simulink model "Longitudinal_fixed_slip"  (R2025b)
settings: Solver=VariableStepAuto  StartTime=0.0  StopTime=5  MaxStep=0.001  RelTol=1e-3
undefined symbols (not defined in the file): car, rad, s, Tau_1, Tau_2, Tau_3, Tau_4, Tau_EM, tyre
libraries: aerolibconvert2 x3, simulink x2
(part 1 of 2)
settings Model: Creator=mzacc  LastModifiedBy=loren

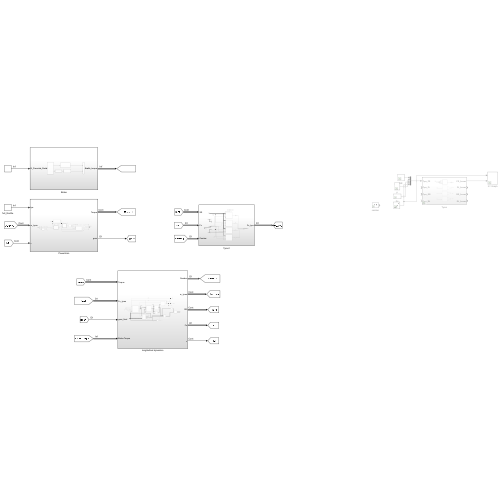
[thumbnail: Simulink's stored preview of the top-level diagram]
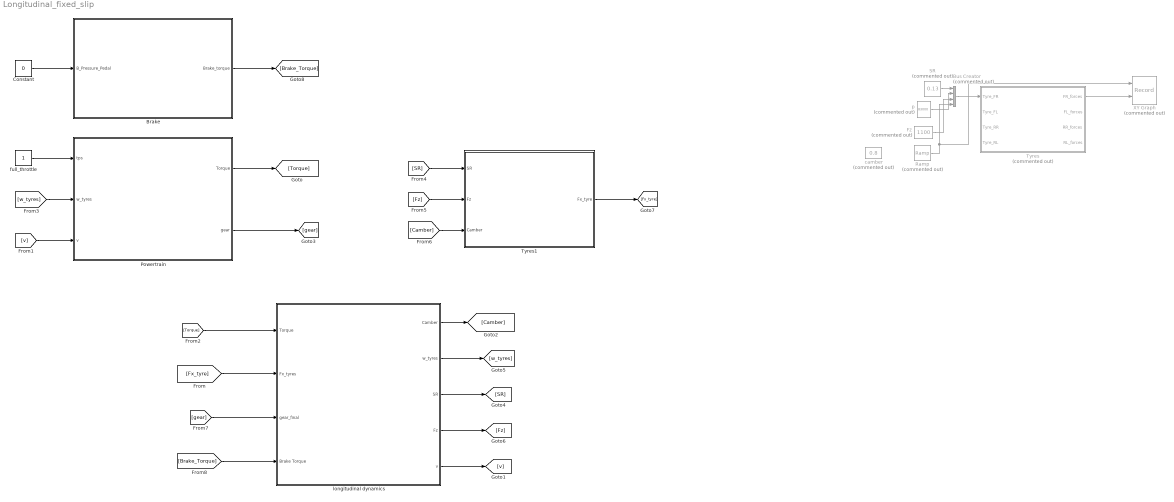
== system Longitudinal_fixed_slip ==
  Brake : Subsystem
  Bus Creator : BusCreator  Commented=on  Inputs=4
  Constant : Constant  Value=0
  Fz : Constant  Commented=on  Value=1100
  Powertrain : Subsystem
  Ramp : simulink/Sources/Ramp  Commented=on  slope=0.05  start=0  InitialOutput=-3
  SR : Constant  Commented=on  Value=0.13
  Tyres : Subsystem  Commented=on
  Tyres1 : Subsystem
  XY Graph : Record  Commented=on  NumPorts=2.0  FileSettingsInternal="{\"entries\":[{\"content\":{\"excelSettings\":{\"content\":{},\"type\":\"Streamout.ExcelSettings\"},\"parquetSettings\":{\"content\":{},\"type\":\"Streamout.ParquetSettings\"}},\"type\":\"Streamout.FileSettingStorage\",\"uuid\":\"\"}],\"packageUris\":[\"http:\\/\\/schema.mathworks.com\\/mf0\\/streamout_blocks\\/R2020a\"],\"version\":\"1.0\"}"  FrameSettings=[0, 0]  Layout=[1 1]  SignalsInternal="{\"entries\":[{\"content\":{},\"type\":\"RecordBlkView.InputSignals\",\"uuid\":\"\"}],\"packageUris\":[\"http:\\/\\/schema.mathworks.com\\/mf0\\/streamout_blocks\\/R2020a\"],\"version\":\"1.0\"}"  VisualizationBindings="{\"xyplotplugin\":{\"info\":[{\"series\":[],\"subplotID\":1}]}}"  CompatibilityTag=XY
  camber : Constant  Commented=on  Value=0.8
  full_throttle : Constant
  longitudinal dynamics : Subsystem
  p : Constant  Commented=on  Value=83000
  wires:
  [Fx_tyre] -> longitudinal dynamics/2(Fx_tyres)
  [Torque] -> longitudinal dynamics/1(Torque)
  Powertrain/1(Torque) -> [Torque]
  Fz/1 -> Bus Creator/3
  Tyres/1(FR_forces) -> XY Graph/2
  p/1 -> Bus Creator/2
  Bus Creator/1 -> Tyres/1(Tyre_FR)
  SR/1 -> Bus Creator/1
  Ramp/1 -> XY Graph/1, Bus Creator/4
  longitudinal dynamics/1(Camber) -> [Camber]
  [w_tyres] -> Powertrain/2(w_tyres)
  longitudinal dynamics/3(SR) -> [SR]
  longitudinal dynamics/2(w_tyres) -> [w_tyres]
  longitudinal dynamics/4(Fz) -> [Fz]
  longitudinal dynamics/5(v) -> [v]
  [v] -> Powertrain/3(v)
  [SR] -> Tyres1/1(SR)
  [Fz] -> Tyres1/2(Fz)
  [Camber] -> Tyres1/3(Camber)
  Tyres1/1(Fx_tyre) -> [Fx_tyre]
  full_throttle/1 -> Powertrain/1(tps)
  Powertrain/2(gear) -> [gear]
  [gear] -> longitudinal dynamics/3(gear_final)
  Constant/1 -> Brake/1(B_Pressure_Pedal)
  Brake/1(Brake_torque) -> [Brake_Torque]
  [Brake_Torque] -> longitudinal dynamics/4(Brake Torque)

== system Longitudinal_fixed_slip/Brake ==
  B_Pressure_Pedal : Inport
  Brake Balance : Subsystem
  Bus Creator : BusCreator  Inputs=2
  Front Caliper : Subsystem
  Proportioning Valve : Subsystem
  Rear Caliper : Subsystem
  Brake_torque : Outport
  wires:
  Brake Balance/1(P_Front) -> Front Caliper/1(P_Front)
  Proportioning Valve/1(p_rear_mod) -> Rear Caliper/1(P_rear)
  Brake Balance/2(P_rear) -> Proportioning Valve/1(P_rear)
  B_Pressure_Pedal/1 -> Brake Balance/1(Braking_Force)
  Bus Creator/1 -> Brake_torque/1
  Front Caliper/1(Brake_torque_front) -> Bus Creator/1  "Brake_torque_front"
  Rear Caliper/1(Brake_torque_rear) -> Bus Creator/2  "Brake_torque_rear"

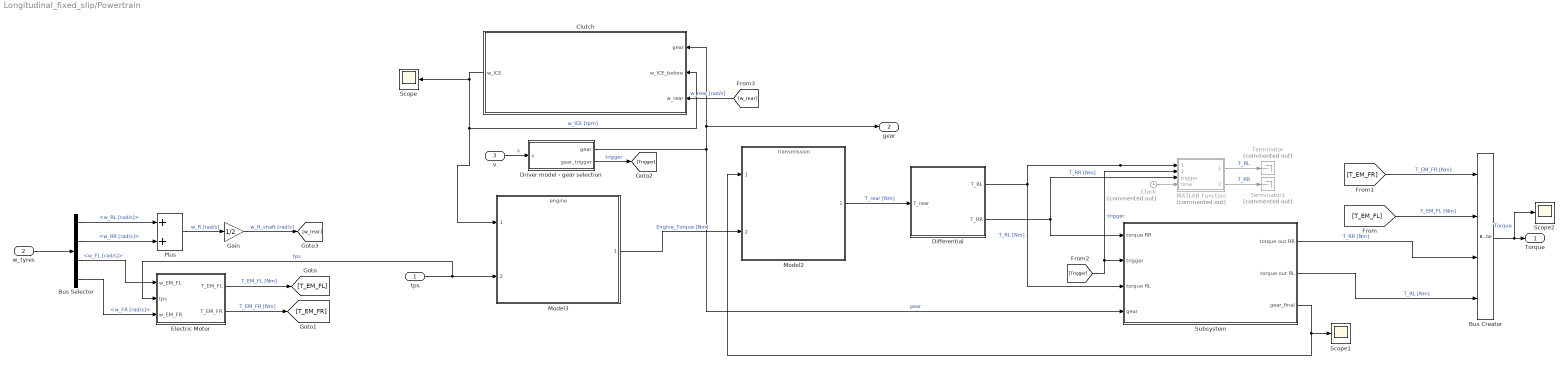
== system Longitudinal_fixed_slip/Powertrain ==
  tps : Inport
  w_tyres : Inport  Port=2
  v : Inport  Port=3
  Bus Creator : BusCreator  Inputs=4
  Bus Selector : BusSelector  OutputSignals=w_RL [rad/s],w_RR [rad/s],w_FL [rad/s],w_FR [rad/s]
  Clock : Clock  Commented=on
  Clutch : Subsystem
  Differential : Subsystem
  Driver model - gear selection : Subsystem
  Electric Motor : Subsystem
  Gain : Gain  Gain=1/2
  MATLAB Function : MATLAB Function  Commented=on  TreatAsAtomicUnit=on
  Model2 : ModelReference  ModelNameDialog=transmission.slx  SimulationMode=Normal  ModelReferenceVersion=3.11
  Model3 : ModelReference  ModelNameDialog=engine.slx  SimulationMode=Normal  ModelReferenceVersion=3.3
  Plus : Sum
  Scope : Scope
      settings: ActiveDisplayYMinimum=5410.5426113045514  ActiveDisplayYMaximum=8668.3318648594359  DataLoggingVariableName=ScopeData5
  Scope1 : Scope
      settings: ActiveDisplayYMinimum=-0.37499999999999989  ActiveDisplayYMaximum=3.375  DataLoggingVariableName=ScopeData4
  Scope2 : Scope
      settings: ActiveDisplayYMinimum=-45.581420561628825  ActiveDisplayYMaximum=410.23278505465947  DataLoggingVariableName=ScopeData19
  Subsystem : Subsystem
  Terminator : Terminator  Commented=on
  Terminator1 : Terminator  Commented=on
  Torque : Outport
  gear : Outport  Port=2
  wires:
  Model3/1 -> Model2/2  "Engine_Torque [Nm]"
  tps/1 -> Electric Motor/2(tps), Model3/2  "tps"
  Model2/1 -> Differential/1(T_rear)  "T_rear [Nm]"
  Bus Creator/1 -> Scope2/1, Torque/1  "Torque"
  Electric Motor/1(T_EM_FL) -> [T_EM_FL]  "T_EM_FL [Nm]"
  Electric Motor/2(T_EM_FR) -> [T_EM_FR]  "T_EM_FR [Nm]"
  [T_EM_FL] -> Bus Creator/2  "T_EM_FL [Nm]"
  [T_EM_FR] -> Bus Creator/1  "T_EM_FR [Nm]"
  Differential/2(T_RR) -> MATLAB Function/3(trigger), Subsystem/1(torque RR)  "T_RR [Nm]"
  Differential/1(T_RL) -> MATLAB Function/1(T_RL_in), Subsystem/3(torque RL)  "T_RL [Nm]"
  Driver model - gear selection/2(gear_trigger) -> [Trigger]  "trigger"
  [Trigger] -> MATLAB Function/2(T_RR_in), Subsystem/2(trigger)  "trigger"
  w_tyres/1 -> Bus Selector/1
  Bus Selector/1 -> Plus/1  "<w_RL [rad/s]>"
  Gain/1 -> [w_rear]  "w_R_shaft [rad/s]"
  Plus/1 -> Gain/1  "w_R [rad/s]"
  Driver model - gear selection/1(gear) -> gear/1, Clutch/1(gear), Subsystem/4(gear)  "gear"
  Clutch/1(w_ICE) -> Model3/1, Clutch/2(w_ICE_before), Scope/1  "w_ICE [rpm]"
  Bus Selector/2 -> Plus/2  "<w_RR [rad/s]>"
  Bus Selector/3 -> Electric Motor/1(w_EM_FL)  "<w_FL [rad/s]>"
  Bus Selector/4 -> Electric Motor/3(w_EM_FR)  "<w_FR [rad/s]>"
  [w_rear] -> Clutch/3(w_rear)  "w_rear [rad/s]"
  v/1 -> Driver model - gear selection/1(v)  "v"
  MATLAB Function/1(T_RL_out) -> Terminator/1  "T_RL"
  MATLAB Function/2(T_RR_out) -> Terminator1/1  "T_RR"
  Clock/1 -> MATLAB Function/4(time)
  Subsystem/1(torque out RR) -> Bus Creator/3  "T_RR [Nm]"
  Subsystem/2(torque out RL) -> Bus Creator/4  "T_RL [Nm]"
  Subsystem/3(gear_final) -> Scope1/1, Model2/1

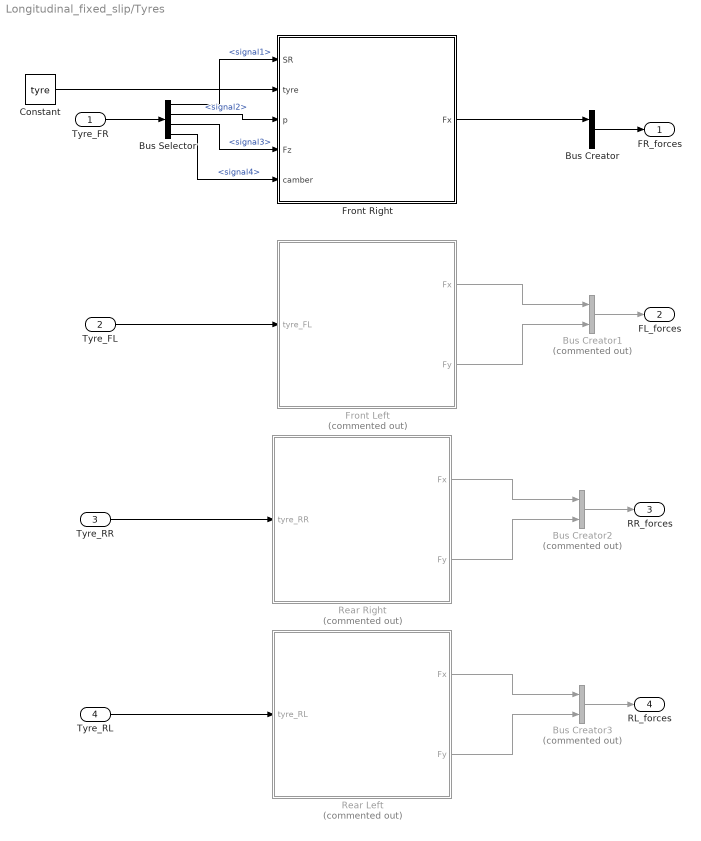
== system Longitudinal_fixed_slip/Tyres ==
  Tyre_FR : Inport
  Tyre_FL : Inport  Port=2
  Tyre_RR : Inport  Port=3
  Tyre_RL : Inport  Port=4
  Bus Creator : BusCreator  Inputs=2
  Bus Creator1 : BusCreator  Commented=on  Inputs=2
  Bus Creator2 : BusCreator  Commented=on  Inputs=2
  Bus Creator3 : BusCreator  Commented=on  Inputs=2
  Bus Selector : BusSelector  OutputSignals=signal1,signal2,signal3,signal4
  Constant : Constant  Value=tyre  OutDataTypeStr=Bus: slBus1
  Front Left : MATLAB Function  Commented=on  TreatAsAtomicUnit=on
  Front Right : MATLAB Function  TreatAsAtomicUnit=on
  Rear Left : MATLAB Function  Commented=on  TreatAsAtomicUnit=on
  Rear Right : MATLAB Function  Commented=on  TreatAsAtomicUnit=on
  FR_forces : Outport
  FL_forces : Outport  Port=2
  RR_forces : Outport  Port=3
  RL_forces : Outport  Port=4
  wires:
  Front Right/1(Fx) -> Bus Creator/1
  Tyre_FL/1 -> Front Left/1(tyre_FL)
  Tyre_RR/1 -> Rear Right/1(tyre_RR)
  Tyre_RL/1 -> Rear Left/1(tyre_RL)
  Bus Creator/1 -> FR_forces/1
  Front Left/1(Fx) -> Bus Creator1/1
  Front Left/2(Fy) -> Bus Creator1/2
  Bus Creator1/1 -> FL_forces/1
  Rear Right/1(Fx) -> Bus Creator2/1
  Rear Right/2(Fy) -> Bus Creator2/2
  Bus Creator2/1 -> RR_forces/1
  Rear Left/1(Fx) -> Bus Creator3/1
  Rear Left/2(Fy) -> Bus Creator3/2
  Bus Creator3/1 -> RL_forces/1
  Tyre_FR/1 -> Bus Selector/1
  Bus Selector/1 -> Front Right/1(SR)  "<signal1>"
  Bus Selector/2 -> Front Right/3(p)  "<signal2>"
  Bus Selector/3 -> Front Right/4(Fz)  "<signal3>"
  Bus Selector/4 -> Front Right/5(camber)  "<signal4>"
  Constant/1 -> Front Right/2(tyre)

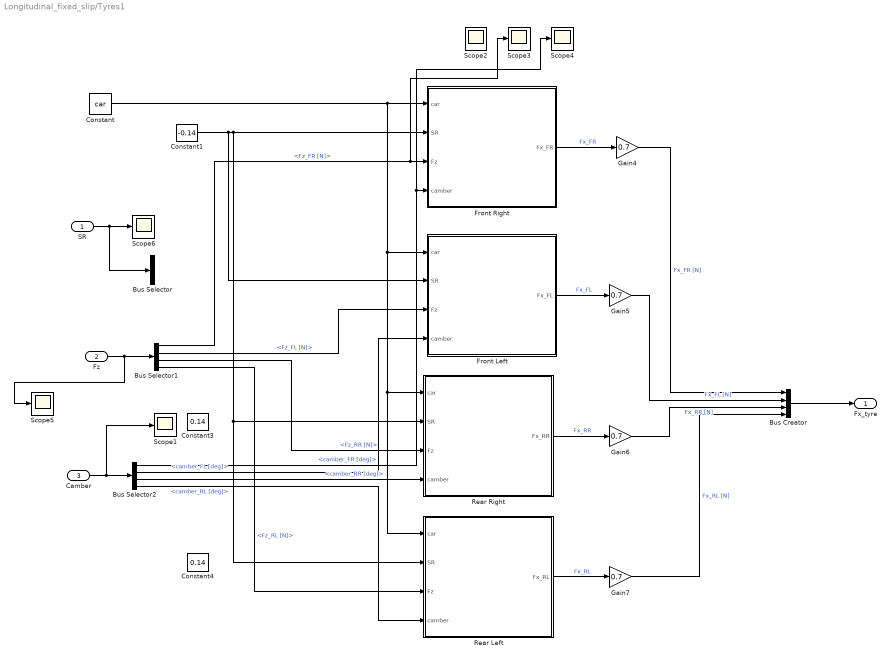
== system Longitudinal_fixed_slip/Tyres1 ==
  SR : Inport
  Fz : Inport  Port=2
  Camber : Inport  Port=3
  Bus Creator : BusCreator  Inputs=4
  Bus Selector : BusSelector  OutputSignals=SR_FL,SR_RL,SR_RR,SR_FR
  Bus Selector1 : BusSelector  OutputSignals=Fz_FR [N],Fz_FL [N],Fz_RR [N],Fz_RL [N]
  Bus Selector2 : BusSelector  OutputSignals=camber_FR [deg],camber_FL [deg],camber_RR [deg],camber_RL [deg]
  Constant : Constant  Value=car  OutDataTypeStr=Bus: slBus1
  Constant1 : Constant  Value=-0.14
  Constant3 : Constant  Value=0.14
  Constant4 : Constant  Value=0.14
  Front Left : MATLAB Function  TreatAsAtomicUnit=on
  Front Right : MATLAB Function  TreatAsAtomicUnit=on
  Gain{4..7} (4 alike) : Gain  Gain=0.7
  Rear Left : MATLAB Function  TreatAsAtomicUnit=on
  Rear Right : MATLAB Function  TreatAsAtomicUnit=on
  Scope{1..6} (6 alike) : Scope
      Scope1 settings: ActiveDisplayYMinimum=-1  ActiveDisplayYMaximum=1  DataLoggingVariableName=ScopeData27
      Scope2 settings: ActiveDisplayYMinimum=-1.2903982949278723  ActiveDisplayYMaximum=0.18800882212526682  DataLoggingVariableName=ScopeData6
      Scope3 settings: ActiveDisplayYMinimum=246.86785737661717  ActiveDisplayYMaximum=1297.36957232489  DataLoggingVariableName=ScopeData7
      Scope4 settings: ActiveDisplayYMinimum=-7.8867077725150958  ActiveDisplayYMaximum=2.0712522631883972  DataLoggingVariableName=ScopeData8
      Scope5 settings: ActiveDisplayYMinimum=-1  ActiveDisplayYMaximum=1  DataLoggingVariableName=ScopeData28
      Scope6 settings: ActiveDisplayYMinimum=-13.029799483705139  ActiveDisplayYMaximum=1.675400103949096  DataLoggingVariableName=ScopeData20
  Fx_tyre : Outport
  wires:
  Constant/1 -> Rear Left/1(car), Rear Right/1(car), Front Left/1(car), Front Right/1(car)
  Bus Creator/1 -> Fx_tyre/1
  Fz/1 -> Scope5/1, Bus Selector1/1
  Camber/1 -> Scope1/1, Bus Selector2/1
  Bus Selector1/1 -> Scope3/1, Front Right/3(Fz)  "<Fz_FR [N]>"
  Bus Selector2/1 -> Scope4/1, Front Right/4(camber)  "<camber_FR [deg]>"
  Bus Selector1/2 -> Front Left/3(Fz)  "<Fz_FL [N]>"
  Bus Selector1/3 -> Rear Right/3(Fz)  "<Fz_RR [N]>"
  Bus Selector1/4 -> Rear Left/3(Fz)  "<Fz_RL [N]>"
  Bus Selector2/2 -> Front Left/4(camber)  "<camber_FL [deg]>"
  Bus Selector2/3 -> Rear Right/4(camber)  "<camber_RR [deg]>"
  Bus Selector2/4 -> Rear Left/4(camber)  "<camber_RL [deg]>"
  SR/1 -> Bus Selector/1, Scope6/1
  Front Right/1(Fx_FR) -> Gain4/1  "Fx_FR"
  Front Left/1(Fx_FL) -> Gain5/1  "Fx_FL"
  Rear Right/1(Fx_RR) -> Gain6/1  "Fx_RR"
  Rear Left/1(Fx_RL) -> Gain7/1  "Fx_RL"
  Gain4/1 -> Bus Creator/1  "Fx_FR [N]"
  Gain5/1 -> Bus Creator/2  "Fx_FL [N]"
  Gain6/1 -> Bus Creator/3  "Fx_RR [N]"
  Gain7/1 -> Bus Creator/4  "Fx_RL [N]"
  Constant1/1 -> Rear Left/2(SR), Rear Right/2(SR), Front Right/2(SR), Front Left/2(SR)

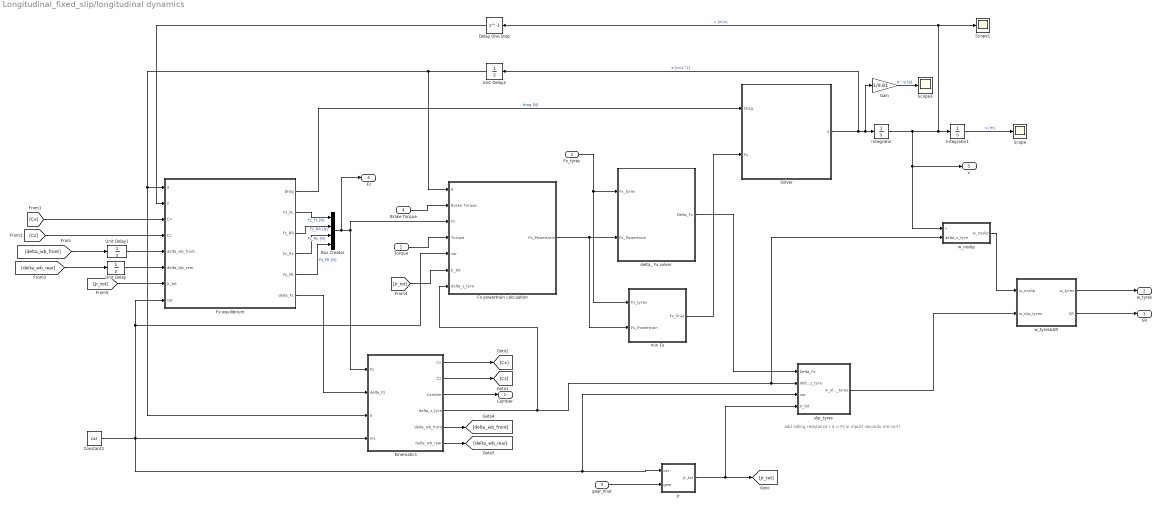
== system Longitudinal_fixed_slip/longitudinal dynamics ==
  note: add rolling resistance ( 4 = Fz in input) secondo me no!!!
  Torque : Inport
  Fx_tyres : Inport  Port=2
  gear_final : Inport  Port=3
  Brake Torque : Inport  Port=4
  Bus Creator : BusCreator  Inputs=4
  Constant1 : Constant  Value=car  OutDataTypeStr=Bus: slBus1
  Delay One Step : Delay  DelayLength=1
  Fx equilibrium : MATLAB Function  TreatAsAtomicUnit=on
  Fx powertrain calculation : Subsystem
  Gain : Gain  Gain=1/9.81
  Integrator : Integrator
  Integrator1 : Integrator
  Jr : Subsystem
  Kinematics : Subsystem
  Scope : Scope
      settings: ActiveDisplayYMinimum=2.4946310045593236  ActiveDisplayYMaximum=116.12903261010605
  Scope1 : Scope
      settings: ActiveDisplayYMinimum=-1  ActiveDisplayYMaximum=1
  Scope3 : Scope
      settings: ActiveDisplayYMinimum=-1.4648722058071688  ActiveDisplayYMaximum=0.89428927320913831  DataLoggingVariableName=ScopeData3
  Solver : Subsystem
  Unit Delay : UnitDelay  SampleTime=-1  HasFrameUpgradeWarning=on
  Unit Delay1 : UnitDelay  SampleTime=-1  HasFrameUpgradeWarning=on
  Unit Delay2 : UnitDelay  SampleTime=-1  HasFrameUpgradeWarning=on
  delta_ Fx solver : Subsystem
  min Fx : Subsystem
  slip_tyres : Subsystem
  w_noslip : Subsystem
  w_tyres&SR : Subsystem
  Camber : Outport
  w_tyres : Outport  Port=2
  SR : Outport  Port=3
  Fz : Outport  Port=4
  v : Outport  Port=5
  wires:
  Torque/1 -> Fx powertrain calculation/4(Torque)
  Integrator1/1 -> Scope/1  "s [m]"
  Integrator/1 -> Delay One Step/1, Scope1/1, Integrator1/1, w_noslip/1(v), v/1  "v [m/s]"
  Fx equilibrium/2(Fz_FL) -> Bus Creator/1  "Fz_FL [N]"
  Fx equilibrium/3(Fz_RR) -> Bus Creator/2  "Fz_RR [N]"
  Fx equilibrium/4(Fz_RL) -> Bus Creator/3  "Fz_RL [N]"
  Fx equilibrium/5(Fz_FR) -> Bus Creator/4  "Fz_FR [N]"
  Bus Creator/1 -> Fz/1, Kinematics/1(Fz), Fx powertrain calculation/3(Fz)
  Fx powertrain calculation/1(Fx_Powertrain) -> min Fx/2(Fx_Powertrain), delta_ Fx solver/2(Fx_Powertrain)
  Fx_tyres/1 -> min Fx/1(Fx_tyres), delta_ Fx solver/1(Fx_tyres)
  delta_ Fx solver/1(Delta_Fx) -> slip_tyres/1(Delta_Fx)
  Kinematics/4(delta_z_tyre) -> Fx powertrain calculation/7(delta_z_tyre), w_noslip/2(delta_z_tyre), slip_tyres/2(delta_z_tyre)
  Kinematics/3(Camber) -> Camber/1
  slip_tyres/1(w_slip_tyres) -> w_tyres&SR/2(w_slip_tyres)
  Fx equilibrium/6(delta_Fz) -> Kinematics/2(delta_Fz)
  Kinematics/2(Cz) -> [Cz]
  Kinematics/1(Cx) -> [Cx]
  [Cx] -> Fx equilibrium/3(Cx)
  [Cz] -> Fx equilibrium/4(Cz)
  Kinematics/5(delta_wb_front) -> [delta_wb_front]
  Kinematics/6(delta_wb_rear) -> [delta_wb_rear]
  [delta_wb_front] -> Unit Delay1/1
  [delta_wb_rear] -> Unit Delay/1
  w_tyres&SR/1(w_tyres) -> w_tyres/1
  w_tyres&SR/2(SR) -> SR/1
  Fx equilibrium/1(Drag) -> Solver/1(Drag)  "drag [N]"
  Delay One Step/1 -> Fx equilibrium/2(v)
  Unit Delay2/1 -> Fx powertrain calculation/1(a), Kinematics/3(a), Fx equilibrium/1(a)
  Constant1/1 -> Jr/1(car), slip_tyres/3(car), Kinematics/4(In1), Fx powertrain calculation/5(car), Fx equilibrium/8(car)
  Unit Delay1/1 -> Fx equilibrium/5(delta_wb_front)
  Solver/1(a) -> Unit Delay2/1, Gain/1, Integrator/1  "a [m/s^2]"
  Gain/1 -> Scope3/1  "a - g [g]"
  w_noslip/1(w_noslip) -> w_tyres&SR/1(w_noslip)
  Unit Delay/1 -> Fx equilibrium/6(delta_wb_rear)
  gear_final/1 -> Jr/2(gear)
  Jr/1(Jr_tot) -> [Jr_tot], slip_tyres/4(Jr_tot)
  [Jr_tot] -> Fx powertrain calculation/6(Jr_tot)
  [Jr_tot] -> Fx equilibrium/7(Jr_tot)
  Brake Torque/1 -> Fx powertrain calculation/2(Brake Torque)
  min Fx/1(Fx_final) -> Solver/2(Fx)

== system Longitudinal_fixed_slip/Brake/Brake Balance ==
  Braking_Force : Inport
  1- Brake_Balance : Gain  Gain=1-car.brakebalance
  Brake_Balance : Gain  Gain=car.brakebalance
  P_Front : Outport
  P_rear : Outport  Port=2
  wires:
  Braking_Force/1 -> Brake_Balance/1, 1- Brake_Balance/1
  1- Brake_Balance/1 -> P_rear/1  "P_rear"
  Brake_Balance/1 -> P_Front/1  "P_Front"

== system Longitudinal_fixed_slip/Brake/Front Caliper ==
  P_Front : Inport
  Gain : Gain  Gain=4
  Pad Friction : Gain  Gain=car.brakepad_friction_coeff
  Piston Area : Gain  Gain=pi*(car.brakepistondiameter)^2/4
  brake radius : Gain  Gain=car.brake_radius_front
  Brake_torque_front : Outport
  wires:
  P_Front/1 -> Gain/1
  Gain/1 -> Piston Area/1
  Piston Area/1 -> Pad Friction/1
  Pad Friction/1 -> brake radius/1
  brake radius/1 -> Brake_torque_front/1

== system Longitudinal_fixed_slip/Brake/Proportioning Valve ==
  P_rear : Inport
  Saturation : Saturate  UpperLimit=car.proportioning_valve_cutting_p  LowerLimit=0
  p_rear_mod : Outport
  wires:
  Saturation/1 -> p_rear_mod/1
  P_rear/1 -> Saturation/1

== system Longitudinal_fixed_slip/Brake/Rear Caliper ==
  P_rear : Inport
  Gain : Gain  Gain=2
  Pad Friction : Gain  Gain=car.brakepad_friction_coeff
  Piston Area : Gain  Gain=pi*(car.brakepistondiameter)^2/4
  brake radius_rear : Gain  Gain=car.brake_radius_rear
  Brake_torque_rear : Outport
  wires:
  Piston Area/1 -> Pad Friction/1
  Gain/1 -> Piston Area/1
  P_rear/1 -> Gain/1
  Pad Friction/1 -> brake radius_rear/1
  brake radius_rear/1 -> Brake_torque_rear/1

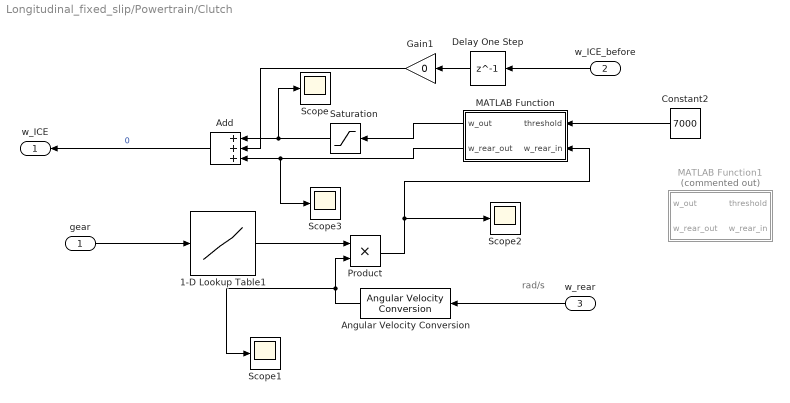
== system Longitudinal_fixed_slip/Powertrain/Clutch ==
  note: rad/s
  gear : Inport
  w_ICE_before : Inport  Port=2
  w_rear : Inport  Port=3
  1-D Lookup Table1 : Lookup_n-D  NumberOfTableDimensions=1  BreakpointsForDimension1=[1;2;3;4]  Table=[Tau_1; Tau_2; Tau_3; Tau_4]  InternalRulePriority=Speed  RndMeth=Simplest
  Add : Sum  Inputs=+++
  Angular Velocity Conversion : aerolibconvert2/Angular Velocity Conversion  IU=rad/s  OU=rpm
  Constant2 : Constant  Value=7000
  Delay One Step : Delay  DelayLength=1
  Gain1 : Gain  Gain=0
  MATLAB Function : MATLAB Function  TreatAsAtomicUnit=on  SystemSampleTime=0.001
  MATLAB Function1 : MATLAB Function  Commented=on  TreatAsAtomicUnit=on  SystemSampleTime=0.001
  Product : Product
  Saturation : Saturate  UpperLimit=10000  LowerLimit=0
  Scope{,1..3} (4 alike) : Scope
      Scope settings: ActiveDisplayYMinimum=-2311.872852964088  ActiveDisplayYMaximum=5444.7682269284924  DataLoggingVariableName=ScopeData9
      Scope1 settings: ActiveDisplayYMinimum=-1  ActiveDisplayYMaximum=1  DataLoggingVariableName=ScopeData16
      Scope2 settings: ActiveDisplayYMinimum=-1232.0255145373203  ActiveDisplayYMaximum=15203.537686190353  DataLoggingVariableName=ScopeData22
      Scope3 settings: ActiveDisplayYMinimum=-5859.3618694424358  ActiveDisplayYMaximum=14721.316107465498  DataLoggingVariableName=ScopeData23
  w_ICE : Outport
  wires:
  Saturation/1 -> Scope/1, Add/1
  MATLAB Function/1(w_out) -> Saturation/1
  w_rear/1 -> Angular Velocity Conversion/1
  1-D Lookup Table1/1 -> Product/1
  Product/1 -> Scope2/1, MATLAB Function/2(w_rear_in)
  Delay One Step/1 -> Gain1/1
  w_ICE_before/1 -> Delay One Step/1
  gear/1 -> 1-D Lookup Table1/1
  Gain1/1 -> Add/2
  Add/1 -> w_ICE/1  "0"
  Angular Velocity Conversion/1 -> Scope1/1, Product/2
  Constant2/1 -> MATLAB Function/1(threshold)
  MATLAB Function/2(w_rear_out) -> Scope3/1, Add/3

== system Longitudinal_fixed_slip/Powertrain/Differential ==
  T_rear : Inport
  Gain : Gain  Gain=0.5
  T_RL : Outport
  T_RR : Outport  Port=2
  wires:
  T_rear/1 -> Gain/1
  Gain/1 -> T_RR/1, T_RL/1

== system Longitudinal_fixed_slip/Powertrain/Driver model - gear selection ==
  v : Inport
  Constant : Constant  Value=car  OutDataTypeStr=Bus: slBus1
  MATLAB Function3 : MATLAB Function  TreatAsAtomicUnit=on
  gear : Outport
  gear_trigger : Outport  Port=2
  wires:
  MATLAB Function3/2(gear_out) -> gear/1
  MATLAB Function3/1(gear_trigger) -> gear_trigger/1  "trigger"
  v/1 -> MATLAB Function3/2(v)
  Constant/1 -> MATLAB Function3/1(car)

== system Longitudinal_fixed_slip/Powertrain/Electric Motor ==
  w_EM_FL : Inport
  tps : Inport  Port=2
  w_EM_FR : Inport  Port=3
  2-D Lookup Table : Lookup_n-D  BreakpointsForDimension1=[0;5415.9399999999996;5455.8699999999999;5494.6300000000001;5524.8000000000002;5801.2200000000003;6194.8599999999997;6620.2799999999997;6996.5;7478.6599999999999;8072.5500000000002;8891.9799999999996;8998.9200000000001;9966.8600000000006;10994.200000000001;11872.6;13016.16;13972.65;15994.85]  BreakpointsForDimension2=[0;0.25;0.29999999999999999;0.34999999999999998;0.40000000000000002;0.45000000000000001;0.5;0.59999999999999998;0.69999999999999996;0.80000000000000004;1]  Table=[0 1.72854705 2.07425646 2.41996587 2.7656752899999999 3.1113846999999999 3.4570941099999999 4.1485129299999999 4.8399317000000002 5.5313505699999999 6.9141880000000002;0 1.72755429 2.0730651500000001 2.4185760100000002 2.7640868599999999 3.10959772 3.4551085800000001 4.1461303000000003 4.8371519999999997 5.5281737299999998 6.9102170000000003;0 1.7172173399999999 2.0606608099999999 2.4041042799999999 2.7475477499999998 3.0909912099999999 3.4344346799999999 4.1213216199999998 4.8082086000000004 5.4950954899999997 6.8688690000000001;0 1.7114327 2.0537192399999999 2.3960057799999999 2.7382923199999998 3.0805788600000001 3.4228654000000001 4.1074384799999999 4.7920116000000004 5.4765846399999996 6.8457309999999998;0 1.7057860899999999 2.0469433100000001 2.3881005200000001 2.72925774 3.0704149599999999 3.4115721799999998 4.0938866100000002 4.7762010000000004 5.45851548 6.8231440000000001;0 1.65353861 1.9842463299999999 2.3149540499999999 2.6456617699999998 2.9763694900000002 3.3070772100000001 3.96849265 4.6299080999999997 5.2913235399999996 6.6141540000000001;0 1.57836584 1.89403901 2.2097121799999999 2.5253853500000001 2.8410585199999998 3.15673168 3.7880780199999999 4.4194243999999996 5.0507707000000002 6.3134629999999996;0 1.5001957400000001 1.80023489 2.10027404 2.4003131899999999 2.7003523399999998 3.0003914800000002 3.6004697800000001 4.2005480999999998 4.8006263699999998 6.0007830000000002;0 1.43080228 1.71696274 2.0031231900000002 2.2892836499999998 2.5754440999999999 2.86160456 3.4339254700000001 4.0062464000000002 4.5785672899999996 5.7232089999999998;0 1.34976662 1.6197199499999999 1.8896732700000001 2.1596266000000002 2.4295799200000001 2.69953325 3.2394398899999999 3.7793464999999999 4.3192531900000004 5.3990660000000004;0 1.24874098 1.49848917 1.74823737 1.99798556 2.24773376 2.4974819500000001 2.9969783400000001 3.4964746999999998 3.9959711200000001 4.9949640000000004;0 1.1245459799999999 1.3494551800000001 1.57436438 1.79927357 2.0241827699999999 2.2490919699999998 2.6989103600000002 3.1487288000000002 3.5985471499999999 4.4981840000000002;0 1.11256427 1.3350771299999999 1.5575899799999999 1.7801028299999999 2.0026156899999998 2.22512854 2.67015425 3.1151800000000001 3.5602056700000002 4.4502569999999997;0 0.98525799000000003 1.18230959 1.3793611800000001 1.5764127800000001 1.7734643800000001 1.9705159800000001 2.3646191700000001 2.7587223999999999 3.1528255600000001 3.9410319999999999;0 0.88127745999999996 1.0575329600000001 1.23378845 1.41004394 1.5862994399999999 1.7625549300000001 2.1150659100000002 2.4675769000000001 2.8200878899999999 3.5251100000000002;0 0.79965012999999996 0.95958014999999997 1.11951018 1.2794402 1.43937023 1.59930025 1.9191602999999999 2.2390203999999998 2.5588804000000001 3.198601;0 0.70417978000000003 0.84501572999999996 0.98585168999999995 1.1266876400000001 1.2675236000000001 1.4083595600000001 1.6900314700000001 1.9717034 2.2533752900000001 2.816719;0 0.63972525999999996 0.76767032000000002 0.89561537000000002 1.0235604199999999 1.15150547 1.2794505300000001 1.5353406300000001 1.7912307000000001 2.0471208399999998 2.5589010000000001;0 0.51010575999999996 0.61212690999999997 0.71414805999999997 0.81616922000000003 0.91819037000000003 1.0202115199999999 1.2242538199999999 1.4282961000000001 1.6323384299999999 2.0404230000000001]  InternalRulePriority=Speed  RndMeth=Simplest
      settings: InputPortMap=u0,u1
  2-D Lookup Table1 : Lookup_n-D  BreakpointsForDimension1=[0;5415.9399999999996;5455.8699999999999;5494.6300000000001;5524.8000000000002;5801.2200000000003;6194.8599999999997;6620.2799999999997;6996.5;7478.6599999999999;8072.5500000000002;8891.9799999999996;8998.9200000000001;9966.8600000000006;10994.200000000001;11872.6;13016.16;13972.65;15994.85]  BreakpointsForDimension2=[0;0.25;0.29999999999999999;0.34999999999999998;0.40000000000000002;0.45000000000000001;0.5;0.59999999999999998;0.69999999999999996;0.80000000000000004;1]  Table=[0 1.72854705 2.07425646 2.41996587 2.7656752899999999 3.1113846999999999 3.4570941099999999 4.1485129299999999 4.8399317000000002 5.5313505699999999 6.9141880000000002;0 1.72755429 2.0730651500000001 2.4185760100000002 2.7640868599999999 3.10959772 3.4551085800000001 4.1461303000000003 4.8371519999999997 5.5281737299999998 6.9102170000000003;0 1.7172173399999999 2.0606608099999999 2.4041042799999999 2.7475477499999998 3.0909912099999999 3.4344346799999999 4.1213216199999998 4.8082086000000004 5.4950954899999997 6.8688690000000001;0 1.7114327 2.0537192399999999 2.3960057799999999 2.7382923199999998 3.0805788600000001 3.4228654000000001 4.1074384799999999 4.7920116000000004 5.4765846399999996 6.8457309999999998;0 1.7057860899999999 2.0469433100000001 2.3881005200000001 2.72925774 3.0704149599999999 3.4115721799999998 4.0938866100000002 4.7762010000000004 5.45851548 6.8231440000000001;0 1.65353861 1.9842463299999999 2.3149540499999999 2.6456617699999998 2.9763694900000002 3.3070772100000001 3.96849265 4.6299080999999997 5.2913235399999996 6.6141540000000001;0 1.57836584 1.89403901 2.2097121799999999 2.5253853500000001 2.8410585199999998 3.15673168 3.7880780199999999 4.4194243999999996 5.0507707000000002 6.3134629999999996;0 1.5001957400000001 1.80023489 2.10027404 2.4003131899999999 2.7003523399999998 3.0003914800000002 3.6004697800000001 4.2005480999999998 4.8006263699999998 6.0007830000000002;0 1.43080228 1.71696274 2.0031231900000002 2.2892836499999998 2.5754440999999999 2.86160456 3.4339254700000001 4.0062464000000002 4.5785672899999996 5.7232089999999998;0 1.34976662 1.6197199499999999 1.8896732700000001 2.1596266000000002 2.4295799200000001 2.69953325 3.2394398899999999 3.7793464999999999 4.3192531900000004 5.3990660000000004;0 1.24874098 1.49848917 1.74823737 1.99798556 2.24773376 2.4974819500000001 2.9969783400000001 3.4964746999999998 3.9959711200000001 4.9949640000000004;0 1.1245459799999999 1.3494551800000001 1.57436438 1.79927357 2.0241827699999999 2.2490919699999998 2.6989103600000002 3.1487288000000002 3.5985471499999999 4.4981840000000002;0 1.11256427 1.3350771299999999 1.5575899799999999 1.7801028299999999 2.0026156899999998 2.22512854 2.67015425 3.1151800000000001 3.5602056700000002 4.4502569999999997;0 0.98525799000000003 1.18230959 1.3793611800000001 1.5764127800000001 1.7734643800000001 1.9705159800000001 2.3646191700000001 2.7587223999999999 3.1528255600000001 3.9410319999999999;0 0.88127745999999996 1.0575329600000001 1.23378845 1.41004394 1.5862994399999999 1.7625549300000001 2.1150659100000002 2.4675769000000001 2.8200878899999999 3.5251100000000002;0 0.79965012999999996 0.95958014999999997 1.11951018 1.2794402 1.43937023 1.59930025 1.9191602999999999 2.2390203999999998 2.5588804000000001 3.198601;0 0.70417978000000003 0.84501572999999996 0.98585168999999995 1.1266876400000001 1.2675236000000001 1.4083595600000001 1.6900314700000001 1.9717034 2.2533752900000001 2.816719;0 0.63972525999999996 0.76767032000000002 0.89561537000000002 1.0235604199999999 1.15150547 1.2794505300000001 1.5353406300000001 1.7912307000000001 2.0471208399999998 2.5589010000000001;0 0.51010575999999996 0.61212690999999997 0.71414805999999997 0.81616922000000003 0.91819037000000003 1.0202115199999999 1.2242538199999999 1.4282961000000001 1.6323384299999999 2.0404230000000001]  InternalRulePriority=Speed  RndMeth=Simplest
      settings: InputPortMap=u0,u1
  Angular Velocity Conversion : aerolibconvert2/Angular Velocity Conversion  IU=rad/s  OU=rpm
  Angular Velocity Conversion1 : aerolibconvert2/Angular Velocity Conversion  IU=rad/s  OU=rpm
  Gain{,1..3} (4 alike) : Gain  Gain=Tau_EM
  Limiter : Saturate  UpperLimit=16000  LowerLimit=0
  Limiter1 : Saturate  UpperLimit=16000  LowerLimit=0
  T_EM_FL : Outport
  T_EM_FR : Outport  Port=2
  wires:
  2-D Lookup Table/1 -> Gain/1
  Gain1/1 -> T_EM_FR/1
  2-D Lookup Table1/1 -> Gain1/1
  Gain/1 -> T_EM_FL/1
  Limiter/1 -> 2-D Lookup Table/1
  Limiter1/1 -> 2-D Lookup Table1/1
  tps/1 -> 2-D Lookup Table1/2, 2-D Lookup Table/2
  w_EM_FL/1 -> Angular Velocity Conversion/1
  w_EM_FR/1 -> Angular Velocity Conversion1/1
  Angular Velocity Conversion/1 -> Gain2/1
  Gain2/1 -> Limiter/1
  Angular Velocity Conversion1/1 -> Gain3/1
  Gain3/1 -> Limiter1/1

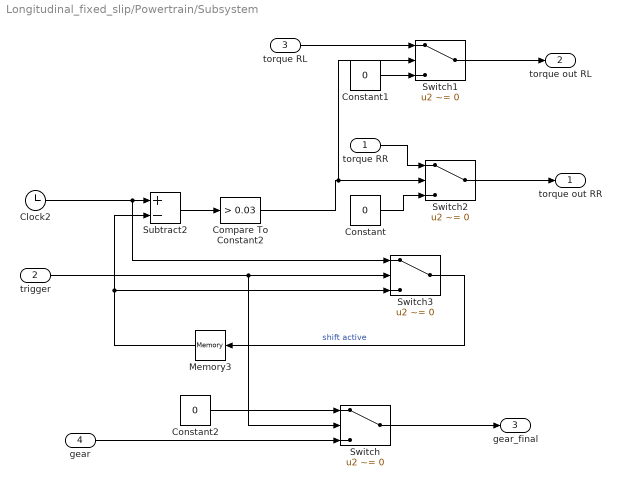
== system Longitudinal_fixed_slip/Powertrain/Subsystem ==
  torque RR : Inport
  trigger : Inport  Port=2
  torque RL : Inport  Port=3
  gear : Inport  Port=4
  Clock2 : Clock
  Compare To Constant2 : simulink/Logic and Bit Operations/Compare To Constant  relop=>  const=0.03  OutDataTypeStr=boolean
  Constant : Constant  Value=0
  Constant1 : Constant  Value=0
  Constant2 : Constant  Value=0
  Memory3 : Memory  InitialCondition=-0.1
  Subtract2 : Sum  Inputs=+-
  Switch{,1..3} (4 alike) : Switch  Criteria=u2 ~= 0  SaturateOnIntegerOverflow=off  InputSameDT=off
  torque out RR : Outport
  torque out RL : Outport  Port=2
  gear_final : Outport  Port=3
  wires:
  Memory3/1 -> Switch3/3, Subtract2/2
  trigger/1 -> Switch/2, Switch3/2
  Switch3/1 -> Memory3/1  "shift active"
  Subtract2/1 -> Compare To Constant2/1
  Switch2/1 -> torque out RR/1
  Switch1/1 -> torque out RL/1
  torque RR/1 -> Switch2/1
  Constant/1 -> Switch2/3
  Constant1/1 -> Switch1/3
  torque RL/1 -> Switch1/1
  Compare To Constant2/1 -> Switch1/2, Switch2/2
  Clock2/1 -> Switch3/1, Subtract2/1
  Constant2/1 -> Switch/1
  gear/1 -> Switch/3
  Switch/1 -> gear_final/1

== system Longitudinal_fixed_slip/longitudinal dynamics/Fx powertrain calculation ==
  a : Inport
  Brake Torque : Inport  Port=2
  Fz : Inport  Port=3
  Torque : Inport  Port=4
  car : Inport  Port=5
  Jr_tot : Inport  Port=6
  delta_z_tyre : Inport  Port=7
  Bus Creator : BusCreator  Inputs=4
  Bus Selector : BusSelector  OutputSignals=T_EM_FL [Nm],T_RR [Nm],T_EM_FR [Nm],T_RL [Nm]
  Bus Selector1 : BusSelector  OutputSignals=Fz_FL [N],Fz_RR [N],Fz_FR [N],Fz_RL [N]
  Bus Selector2 : BusSelector  OutputSignals=Brake_torque_front,Brake_torque_rear
  Bus Selector3 : BusSelector  OutputSignals=delta_z_tyre_FL,delta_z_tyre_RR,delta_z_tyre_FR,delta_z_tyre_RL
  FL : MATLAB Function  TreatAsAtomicUnit=on
  FR : MATLAB Function  TreatAsAtomicUnit=on
  RL : MATLAB Function  TreatAsAtomicUnit=on
  RR : MATLAB Function  TreatAsAtomicUnit=on
  Fx_Powertrain : Outport
  wires:
  FL/1(Fx_EM_FL) -> Bus Creator/1
  RR/1(Fx_ICE_RR) -> Bus Creator/2
  FR/1(Fx_EM_FR) -> Bus Creator/3
  Bus Creator/1 -> Fx_Powertrain/1
  RL/1(Fx_ICE_RL) -> Bus Creator/4
  Torque/1 -> Bus Selector/1
  Bus Selector/1 -> FL/1(T)  "<T_EM_FL [Nm]>"
  Bus Selector/2 -> RR/1(T)  "<T_RR [Nm]>"
  Bus Selector/3 -> FR/1(T)  "<T_EM_FR [Nm]>"
  Bus Selector/4 -> RL/1(T)  "<T_RL [Nm]>"
  Fz/1 -> Bus Selector1/1
  Bus Selector1/1 -> FL/3(Fz)  "<Fz_FL [N]>"
  Bus Selector1/2 -> RR/4(Fz)  "<Fz_RR [N]>"
  Bus Selector1/3 -> FR/3(Fz)  "<Fz_FR [N]>"
  Bus Selector1/4 -> RL/3(Fz)  "<Fz_RL [N]>"
  a/1 -> FL/4(a), RR/3(a), FR/4(a), RL/4(a)
  car/1 -> RL/6(car), FR/5(car), RR/6(car), FL/5(car)
  Jr_tot/1 -> RL/5(J_r), RR/5(J_r)
  Brake Torque/1 -> Bus Selector2/1
  Bus Selector2/1 -> FR/2(T_b), FL/2(T_b)  "<Brake_torque_front>"
  Bus Selector2/2 -> RL/2(T_b), RR/2(T_b)  "<Brake_torque_rear>"
  delta_z_tyre/1 -> Bus Selector3/1
  Bus Selector3/1 -> FL/6(delta_z_tyre_FL)  "<delta_z_tyre_FL>"
  Bus Selector3/2 -> RR/7(delta_z_tyre_RR)  "<delta_z_tyre_RR>"
  Bus Selector3/3 -> FR/6(delta_z_tyre_FR)  "<delta_z_tyre_FR>"
  Bus Selector3/4 -> RL/7(delta_z_tyre_RL)  "<delta_z_tyre_RL>"

== system Longitudinal_fixed_slip/longitudinal dynamics/Jr ==
  car : Inport
  gear : Inport  Port=2
  MATLAB Function : MATLAB Function  TreatAsAtomicUnit=on
  Jr_tot : Outport
  wires:
  gear/1 -> MATLAB Function/1(gear)
  car/1 -> MATLAB Function/2(car)
  MATLAB Function/1(Jr_tot) -> Jr_tot/1

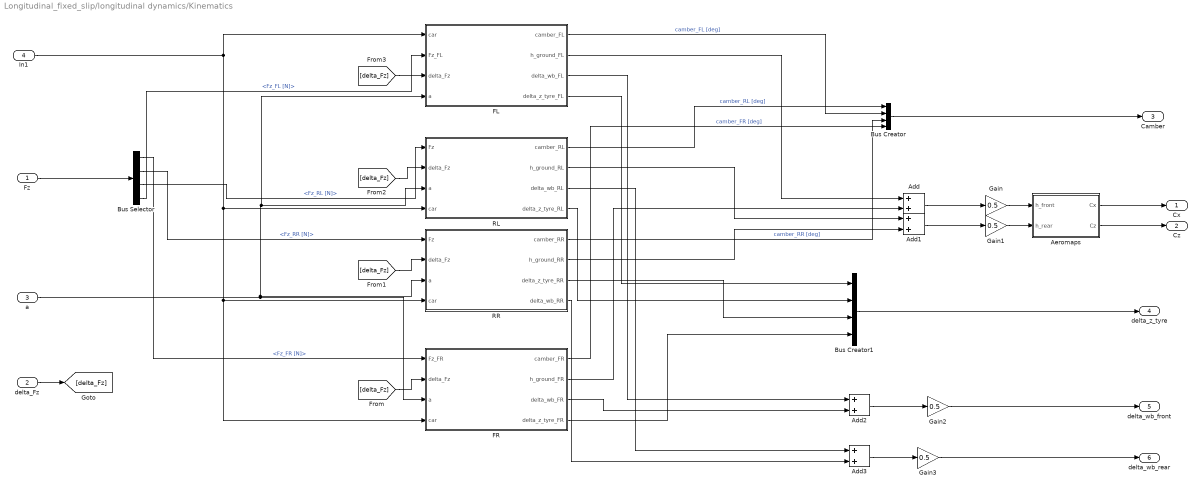
== system Longitudinal_fixed_slip/longitudinal dynamics/Kinematics ==
  Fz : Inport
  delta_Fz : Inport  Port=2
  a : Inport  Port=3
  In1 : Inport  Port=4
  Add{,1..3} (4 alike) : Sum
  Aeromaps : Subsystem
  Bus Creator : BusCreator  Inputs=4
  Bus Creator1 : BusCreator  Inputs=4
  Bus Selector : BusSelector  OutputSignals=Fz_FR [N],Fz_RR [N],Fz_RL [N],Fz_FL [N]
  FL : Subsystem
  FR : Subsystem
  Gain{,1..3} (4 alike) : Gain  Gain=0.5
  RL : Subsystem
  RR : Subsystem
  Cx : Outport
  Cz : Outport  Port=2
  Camber : Outport  Port=3
  delta_z_tyre : Outport  Port=4
  delta_wb_front : Outport  Port=5
  delta_wb_rear : Outport  Port=6
  wires:
  Aeromaps/1(Cx) -> Cx/1
  Aeromaps/2(Cz) -> Cz/1
  RR/1(camber_RR) -> Bus Creator/3  "camber_RR [deg]"
  FR/1(camber_FR) -> Bus Creator/4  "camber_FR [deg]"
  RL/1(camber_RL) -> Bus Creator/1  "camber_RL [deg]"
  Bus Creator/1 -> Camber/1
  Fz/1 -> Bus Selector/1
  Bus Selector/1 -> FR/1(Fz_FR)  "<Fz_FR [N]>"
  Bus Selector/2 -> RR/1(Fz)  "<Fz_RR [N]>"
  Bus Selector/3 -> RL/1(Fz)  "<Fz_RL [N]>"
  [delta_Fz] -> FR/2(delta_Fz)
  [delta_Fz] -> RR/2(delta_Fz)
  [delta_Fz] -> RL/2(delta_Fz)
  Bus Creator1/1 -> delta_z_tyre/1
  RR/3(delta_z_tyre_RR) -> Bus Creator1/3
  delta_Fz/1 -> [delta_Fz]
  FL/1(camber_FL) -> Bus Creator/2  "camber_FL [deg]"
  FL/4(delta_z_tyre_FL) -> Bus Creator1/1
  [delta_Fz] -> FL/3(delta_Fz)
  Bus Selector/4 -> FL/2(Fz_FL)  "<Fz_FL [N]>"
  FR/4(delta_z_tyre_FR) -> Bus Creator1/4
  Add/1 -> Gain/1
  Gain/1 -> Aeromaps/1(h_front)
  FL/2(h_ground_FL) -> Add/1
  FR/2(h_ground_FR) -> Add/2
  Add1/1 -> Gain1/1
  Gain1/1 -> Aeromaps/2(h_rear)
  RR/2(h_ground_RR) -> Add1/2
  RL/2(h_ground_RL) -> Add1/1
  RL/4(delta_z_tyre_RL) -> Bus Creator1/2
  Add2/1 -> Gain2/1
  Gain2/1 -> delta_wb_front/1
  Add3/1 -> Gain3/1
  Gain3/1 -> delta_wb_rear/1
  FR/3(delta_wb_FR) -> Add2/2
  FL/3(delta_wb_FL) -> Add2/1
  RR/4(delta_wb_RR) -> Add3/2
  RL/3(delta_wb_RL) -> Add3/1
  a/1 -> FL/4(a), RL/3(a), RR/3(a), FR/3(a)
  In1/1 -> FR/4(car), RR/4(car), RL/4(car), FL/1(car)

== system Longitudinal_fixed_slip/longitudinal dynamics/Solver ==
  Drag : Inport
  Fx : Inport  Port=2
  Add : Sum  Inputs=++++
  Bus Selector : BusSelector  OutputSignals=Fx_RR [N],Fx_RL [N],Fx_FR [N],Fx_FL [N]
  Gain : Gain  Gain=1/car.m
  Subtract : Sum  Inputs=+-
  a : Outport
  wires:
  Add/1 -> Subtract/1  "Fx total [N]"
  Subtract/1 -> Gain/1
  Drag/1 -> Subtract/2
  Gain/1 -> a/1  "a"
  Fx/1 -> Bus Selector/1
  Bus Selector/1 -> Add/1  "<Fx_RR [N]>"
  Bus Selector/2 -> Add/2  "<Fx_RL [N]>"
  Bus Selector/3 -> Add/3  "<Fx_FR [N]>"
  Bus Selector/4 -> Add/4  "<Fx_FL [N]>"

== system Longitudinal_fixed_slip/longitudinal dynamics/delta_ Fx solver ==
  Fx_tyres : Inport
  Fx_Powertrain : Inport  Port=2
  Bus Creator1 : BusCreator  Inputs=4
  Bus Selector : BusSelector  OutputSignals=Fx_ICE_RR,Fx_ICE_RL,Fx_EM_FL,Fx_EM_FR
  Bus Selector1 : BusSelector  OutputSignals=Fx_RL [N],Fx_RR [N],Fx_FR [N],Fx_FL [N]
  FL : MATLAB Function  TreatAsAtomicUnit=on
  FR : MATLAB Function  TreatAsAtomicUnit=on
  RL : MATLAB Function  TreatAsAtomicUnit=on
  RR : MATLAB Function  TreatAsAtomicUnit=on
  Delta_Fx : Outport
  wires:
  Fx_Powertrain/1 -> Bus Selector/1
  Fx_tyres/1 -> Bus Selector1/1
  Bus Selector/1 -> RR/1(Fx_ICE)  "<Fx_ICE_RR>"
  Bus Selector1/1 -> RL/2(Fx_tyre)  "<Fx_RL [N]>"
  Bus Selector1/2 -> RR/2(Fx_tyre)  "<Fx_RR [N]>"
  Bus Selector/2 -> RL/1(Fx_ICE)  "<Fx_ICE_RL>"
  Bus Selector1/4 -> FL/2(Fx_tyre)  "<Fx_FL [N]>"
  Bus Selector1/3 -> FR/2(Fx_tyre)  "<Fx_FR [N]>"
  Bus Selector/4 -> FR/1(Fx_EM)  "<Fx_EM_FR>"
  Bus Selector/3 -> FL/1(Fx_EM)  "<Fx_EM_FL>"
  Bus Creator1/1 -> Delta_Fx/1
  RR/1(delta_Fx_RR) -> Bus Creator1/1
  RL/1(delta_Fx_RL) -> Bus Creator1/2
  FR/1(delta_Fx_FR) -> Bus Creator1/3
  FL/1(delta_Fx_FL) -> Bus Creator1/4

== system Longitudinal_fixed_slip/longitudinal dynamics/min Fx ==
  Fx_tyres : Inport
  Fx_Powertrain : Inport  Port=2
  Bus Creator : BusCreator  Inputs=4
  Bus Selector : BusSelector  OutputSignals=Fx_FR [N],Fx_FL [N],Fx_RR [N],Fx_RL [N]
  Bus Selector1 : BusSelector  OutputSignals=Fx_ICE_RL,Fx_EM_FR,Fx_ICE_RR,Fx_EM_FL
  Min{,1..3} (4 alike) : MinMax  Inputs=2
  Scope : Scope
      settings: ActiveDisplayYMinimum=-299.65473155083509  ActiveDisplayYMaximum=1256.3160141196672  DataLoggingVariableName=ScopeData10
  Fx_final : Outport
  wires:
  Fx_tyres/1 -> Bus Selector/1
  Fx_Powertrain/1 -> Bus Selector1/1
  Bus Selector/1 -> Min/1  "<Fx_FR [N]>"
  Bus Selector1/1 -> Min2/2  "<Fx_ICE_RL>"
  Bus Selector1/2 -> Min/2  "<Fx_EM_FR>"
  Min/1 -> Bus Creator/1  "Fx_FR [N]"
  Bus Selector/2 -> Min1/1  "<Fx_FL [N]>"
  Bus Selector1/3 -> Min3/2  "<Fx_ICE_RR>"
  Bus Selector1/4 -> Min1/2  "<Fx_EM_FL>"
  Bus Selector/3 -> Min3/1  "<Fx_RR [N]>"
  Bus Selector/4 -> Min2/1  "<Fx_RL [N]>"
  Min1/1 -> Bus Creator/2  "Fx_FL [N]"
  Min2/1 -> Bus Creator/3  "Fx_RL [N]"
  Min3/1 -> Scope/1, Bus Creator/4  "Fx_RR [N]"
  Bus Creator/1 -> Fx_final/1

== system Longitudinal_fixed_slip/longitudinal dynamics/slip_tyres ==
  note: Add rolling resistance
  note: rad/s
  note: [m]
  note: [mm]
  Delta_Fx : Inport
  delta_z_tyre : Inport  Port=2
  car : Inport  Port=3
  Jr_tot : Inport  Port=4
  Bus Creator : BusCreator  Inputs=4
  Bus Selector : BusSelector  OutputSignals=delta_Fx_RR,delta_Fx_RL,delta_Fx_FR,delta_Fx_FL
  Bus Selector1 : BusSelector  OutputSignals=delta_z_tyre_FL,delta_z_tyre_RL,delta_z_tyre_FR,delta_z_tyre_RR
  FL : MATLAB Function  TreatAsAtomicUnit=on
  FR : MATLAB Function  TreatAsAtomicUnit=on
  Integrator{,1..3} (4 alike) : Integrator
  RL : MATLAB Function  TreatAsAtomicUnit=on
  RR : MATLAB Function  TreatAsAtomicUnit=on
  w_slip_tyres : Outport
  wires:
  Delta_Fx/1 -> Bus Selector/1
  Bus Selector/1 -> RR/1(delta_Fx_rear)  "<delta_Fx_RR>"
  Bus Selector/2 -> RL/1(delta_Fx_rear)  "<delta_Fx_RL>"
  Bus Selector/3 -> FR/1(delta_Fx_front)  "<delta_Fx_FR>"
  Bus Selector/4 -> FL/1(delta_Fx_front)  "<delta_Fx_FL>"
  Bus Creator/1 -> w_slip_tyres/1
  FR/1(w_dot_slip_FR) -> Integrator/1  "w_dot_slip_FR"
  Integrator/1 -> Bus Creator/4  "w_slip_FR [rad/s]"
  FL/1(w_dot_slip_FL) -> Integrator1/1
  Integrator1/1 -> Bus Creator/1  "w_slip_FL [rad/s]"
  RR/1(w_dot_slip_RR) -> Integrator2/1  "w_dot_slip_RR"
  Integrator2/1 -> Bus Creator/3  "w_slip_RR [rad/s]"
  RL/1(w_dot_slip_RL) -> Integrator3/1
  Integrator3/1 -> Bus Creator/2  "w_slip_RL [rad/s]"
  Bus Selector1/2 -> RL/2(delta_z_tyre_RL)  "<delta_z_tyre_RL>"
  Bus Selector1/1 -> FL/2(delta_z_tyre_FL)  "<delta_z_tyre_FL>"
  Bus Selector1/3 -> FR/2(delta_z_tyre_FR)  "<delta_z_tyre_FR>"
  Bus Selector1/4 -> RR/2(delta_z_tyre_RR)  "<delta_z_tyre_RR>"
  car/1 -> RL/4(car), FL/3(car), FR/3(car), RR/4(car)
  delta_z_tyre/1 -> Bus Selector1/1
  Jr_tot/1 -> RL/3(J_r), RR/3(J_r)

== system Longitudinal_fixed_slip/longitudinal dynamics/w_noslip ==
  v : Inport
  delta_z_tyre : Inport  Port=2
  Add{,1..3} (4 alike) : Sum  Inputs=+-
  Bus Creator : BusCreator  Inputs=4
  Bus Selector : BusSelector  OutputSignals=delta_z_tyre_RR,delta_z_tyre_RL,delta_z_tyre_FL,delta_z_tyre_FR
  Constant : Constant  Value=car.R
  Divide{,1..3} (4 alike) : Product  Inputs=*/
  Gain{,1..3} (4 alike) : Gain  Gain=0.5
  w_noslip : Outport
  wires:
  Gain1/1 -> Add1/2
  Constant/1 -> Add3/1, Add2/1, Add1/1, Add/1
  Gain2/1 -> Add2/2
  Bus Selector/1 -> Gain/1  "<delta_z_tyre_RR>"
  delta_z_tyre/1 -> Bus Selector/1
  Divide1/1 -> Bus Creator/2  "w_noslip_RL"
  Divide3/1 -> Bus Creator/4  "w_noslip_FR"
  Add/1 -> Divide/2
  Divide2/1 -> Bus Creator/3  "w_noslip_FL"
  Bus Selector/3 -> Gain2/1  "<delta_z_tyre_FL>"
  v/1 -> Divide3/1, Divide2/1, Divide1/1, Divide/1
  Add1/1 -> Divide1/2
  Bus Selector/2 -> Gain1/1  "<delta_z_tyre_RL>"
  Bus Selector/4 -> Gain3/1  "<delta_z_tyre_FR>"
  Bus Creator/1 -> w_noslip/1  "w_noslip"
  Gain3/1 -> Add3/2
  Gain/1 -> Add/2
  Divide/1 -> Bus Creator/1  "w_noslip_RR"
  Add2/1 -> Divide2/2
  Add3/1 -> Divide3/2

== system Longitudinal_fixed_slip/longitudinal dynamics/w_tyres&SR ==
  note: rad/s
  w_noslip : Inport
  w_slip_tyres : Inport  Port=2
  Bus Creator : BusCreator  Inputs=4
  Bus Creator1 : BusCreator  Inputs=4
  Bus Selector : BusSelector  OutputSignals=w_slip_FL [rad/s],w_slip_RL [rad/s],w_slip_RR [rad/s],w_slip_FR [rad/s]
  Bus Selector1 : BusSelector  OutputSignals=w_noslip_FL,w_noslip_RL,w_noslip_RR,w_noslip_FR
  FL : Subsystem
  FR : Subsystem
  RL : Subsystem
  RR : Subsystem
  w_tyres : Outport
  SR : Outport  Port=2
  wires:
  w_slip_tyres/1 -> Bus Selector/1
  Bus Selector/1 -> FL/2(<w_slip_FL>)  "<w_slip_FL [rad/s]>"
  Bus Selector/2 -> RL/2(<w_slip_RL>)  "<w_slip_RL [rad/s]>"
  Bus Selector/3 -> RR/2(<w_slip_RR>)  "<w_slip_RR [rad/s]>"
  Bus Selector/4 -> FR/2(<w_slip_FR>)  "<w_slip_FR [rad/s]>"
  Bus Creator/1 -> w_tyres/1
  FL/1(w_FL) -> Bus Creator/1  "w_FL [rad/s]"
  RL/1(w_RL) -> Bus Creator/2  "w_RL [rad/s]"
  RR/1(w_RR) -> Bus Creator/3  "w_RR [rad/s]"
  FR/1(w_FR) -> Bus Creator/4  "w_FR [rad/s]"
  FL/2(SR_FL) -> Bus Creator1/1  "SR_FL"
  RL/2(SR_RL) -> Bus Creator1/2  "SR_RL"
  RR/2(SR_RR) -> Bus Creator1/3  "SR_RR"
  FR/2(SR_FR) -> Bus Creator1/4  "SR_FR"
  Bus Creator1/1 -> SR/1
  w_noslip/1 -> Bus Selector1/1
  Bus Selector1/1 -> FL/1(w_noslip)  "<w_noslip_FL>"
  Bus Selector1/2 -> RL/1(w_noslip)  "<w_noslip_RL>"
  Bus Selector1/3 -> RR/1(w_noslip)  "<w_noslip_RR>"
  Bus Selector1/4 -> FR/1(w_noslip)  "<w_noslip_FR>"

== system Longitudinal_fixed_slip/longitudinal dynamics/Kinematics/Aeromaps ==
  h_front : Inport
  h_rear : Inport  Port=2
  Constant : Constant  Value=car.Cx
  Constant1 : Constant  Value=car.Cz
  Terminator : Terminator
  Terminator1 : Terminator
  Cx : Outport
  Cz : Outport  Port=2
  wires:
  h_front/1 -> Terminator/1
  h_rear/1 -> Terminator1/1
  Constant/1 -> Cx/1
  Constant1/1 -> Cz/1

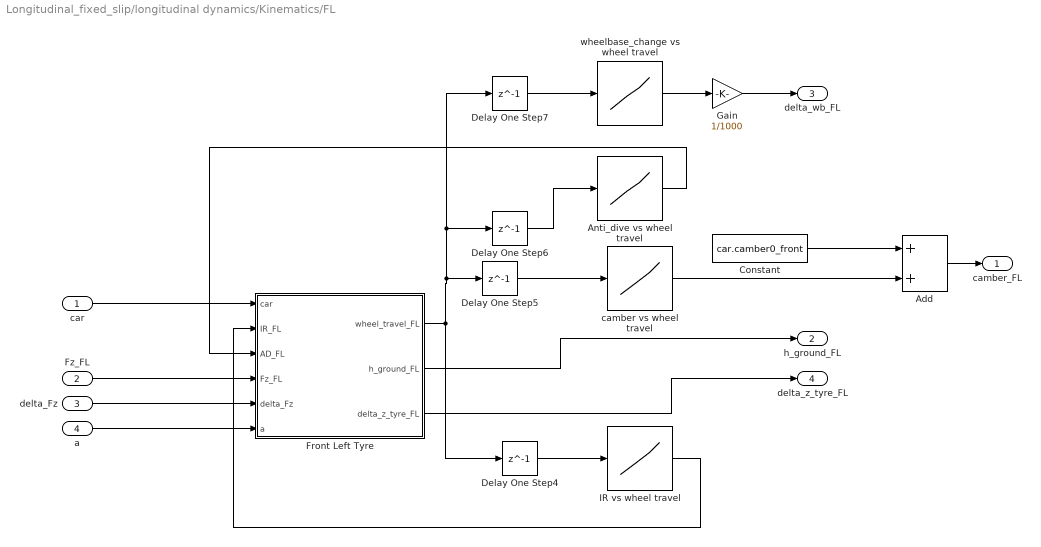
== system Longitudinal_fixed_slip/longitudinal dynamics/Kinematics/FL ==
  car : Inport
  Fz_FL : Inport  Port=2
  delta_Fz : Inport  Port=3
  a : Inport  Port=4
  Add : Sum
  Anti_dive vs wheel travel : Lookup_n-D  NumberOfTableDimensions=1  BreakpointsForDimension1=[-20;-19;-18;-17;-16;-15;-14;-13;-12;-11;-10;-9;-8;-7;-6;-5;-4;-3;-2;-1;0;1;2;3;4;5;6;7;8;9;10;11;12;13;14;15;16;17;18;19;20;21;22;23;24;25;26;27;28;29;30;31;32;33;34;35;36;37;38;39;40;41;42;43;44;45;46;47;48;49;50;51;52;53;54;55;56;57;58;59;60;61;62;63;64;65;66;67;68;69;70;71;72;73;74;75]  Table=[56.11;56.3;56.5;56.69;56.89;57.08;57.28;57.48;57.68;57.88;58.09;58.29;58.5;58.7;58.91;59.12;59.33;59.54;59.76;59.97;60.19;60.4;60.62;60.84;61.06;61.29;61.51;61.74;61.96;62.19;62.42;62.65;62.88;63.12;63.35;63.59;63.83;64.06999999999999;64.31;64.56;64.8;65.05;65.3;65.55;65.8;66.05;66.31;66.56999999999999;66.83;67.09;67.34999999999999;67.61;67.88;68.15000000000001;68.42;68.69;68.95999999999999;69.23999999999999;69.52;69.8;70.08;70.36;70.65000000000001;70.94;71.23;71.52;71.81;72.11;72.41;72.70999999999999;73.02;73.31999999999999;73.63;73.94;74.25;74.56999999999999;74.89;75.20999999999999;75.53;75.84999999999999;76.18000000000001;76.51000000000001;76.84999999999999;77.18000000000001;77.52;77.86;78.20999999999999;78.55;78.90000000000001;79.26000000000001;79.61;79.97;80.33;80.7;81.06;81.43000000000001]  InternalRulePriority=Speed  RndMeth=Simplest
  Constant : Constant  Value=car.camber0_front
  Delay One Step{4..7} (4 alike) : Delay  DelayLength=1
  Front Left Tyre : MATLAB Function  TreatAsAtomicUnit=on
  Gain : Gain  Gain=1/1000
  IR vs wheel travel : Lookup_n-D  NumberOfTableDimensions=1  BreakpointsForDimension1=[-20;-19;-18;-17;-16;-15;-14;-13;-12;-11;-10;-9;-8;-7;-6;-5;-4;-3;-2;-1;0;1;2;3;4;5;6;7;8;9;10;11;12;13;14;15;16;17;18;19;20;21;22;23;24;25;26;27;28;29;30;31;32;33;34;35;36;37;38;39;40;41;42;43;44;45;46;47;48;49;50;51;52;53;54;55;56;57;58;59;60;61;62;63;64;65;66;67;68;69;70;71;72;73;74;75]  Table=[0.5620000000000001;0.562105263157895;0.562222222222222;0.5623529411764711;0.5625;0.562666666666667;0.5628571428571429;0.563076923076923;0.563333333333333;0.562727272727273;0.5629999999999999;0.563333333333333;0.5625;0.5628571428571429;0.563333333333333;0.5639999999999999;0.5625;0.563333333333333;0.5649999999999999;0.5600000000000001;0.5600000000000001;0.5600000000000001;0.5649999999999999;0.563333333333333;0.5625;0.5620000000000001;0.561666666666667;0.5614285714285711;0.56125;0.561111111111111;0.5610000000000001;0.560909090909091;0.560833333333333;0.560769230769231;0.5607142857142861;0.560666666666667;0.5600000000000001;0.5600000000000001;0.559444444444444;0.559473684210526;0.5590000000000001;0.559047619047619;0.558636363636364;0.558260869565217;0.5579166666666669;0.5576;0.5573076923076919;0.557037037037037;0.556785714285714;0.556551724137931;0.556333333333333;0.555806451612903;0.555625;0.555151515151515;0.554705882352941;0.554571428571429;0.554166666666667;0.553783783783784;0.553421052631579;0.553076923076923;0.55275;0.5524390243902439;0.551904761904762;0.551627906976744;0.551136363636364;0.550888888888889;0.550434782608696;0.55;0.549583333333333;0.549183673469388;0.5488;0.54843137254902;0.548076923076923;0.547547169811321;0.5472222222222221;0.546727272727273;0.546428571428571;0.545964912280702;0.54551724137931;0.545084745762712;0.544666666666667;0.544262295081967;0.543870967741935;0.543492063492063;0.543125;0.5426153846153851;0.542272727272727;0.5417910447761189;0.541323529411765;0.587971014492754;0.585285714285714;0.582676056338028;0.580277777777778;0.577808219178082;0.575405405405405;0.5732]  InternalRulePriority=Speed  RndMeth=Simplest
  camber vs wheel travel : Lookup_n-D  NumberOfTableDimensions=1  BreakpointsForDimension1=[-20;-19;-18;-17;-16;-15;-14;-13;-12;-11;-10;-9;-8;-7;-6;-5;-4;-3;-2;-1;0;1;2;3;4;5;6;7;8;9;10;11;12;13;14;15;16;17;18;19;20;21;22;23;24;25;26;27;28;29;30;31;32;33;34;35;36;37;38;39;40;41;42;43;44;45;46;47;48;49;50;51;52;53;54;55;56;57;58;59;60;61;62;63;64;65;66;67;68;69;70;71;72;73;74;75]  Table=[0.94910000000000005;0.90229999999999999;0.85550000000000004;0.80859999999999999;0.76160000000000005;0.71450000000000002;0.66739999999999999;0.62019999999999997;0.57299999999999995;0.52569999999999995;0.4783;0.43080000000000002;0.38319999999999999;0.33560000000000001;0.28789999999999999;0.24010000000000001;0.1923;0.14430000000000001;0.096299999999999997;0.0482;0;-0.048300000000000003;-0.096600000000000005;-0.14510000000000001;-0.19359999999999999;-0.2422;-0.29089999999999999;-0.3397;-0.3886;-0.43759999999999999;-0.48670000000000002;-0.53580000000000005;-0.58509999999999995;-0.63439999999999996;-0.68389999999999995;-0.73340000000000005;-0.78310000000000002;-0.83279999999999998;-0.88270000000000004;-0.93259999999999998;-0.98270000000000002;-1.0327999999999999;-1.0831;-1.1334;-1.1839;-1.2344999999999999;-1.2851999999999999;-1.3360000000000001;-1.3869;-1.4379;-1.4890000000000001;-1.5403;-1.5915999999999999;-1.6431;-1.6947000000000001;-1.7464;-1.7982;-1.8501000000000001;-1.9021999999999999;-1.9543999999999999;-2.0066999999999999;-2.0590999999999999;-2.1116999999999999;-2.1644000000000001;-2.2172000000000001;-2.2700999999999998;-2.3231999999999999;-2.3763999999999998;-2.4297;-2.4830999999999999;-2.5367000000000002;-2.5903999999999998;-2.6442999999999999;-2.6983000000000001;-2.7524000000000002;-2.8067000000000002;-2.8611;-2.9156;-2.9702999999999999;-3.0251000000000001;-3.0800999999999998;-3.1352000000000002;-3.1903999999999999;-3.2458;-3.3014000000000001;-3.3571;-3.4129;-3.4689000000000001;-3.5251000000000001;-3.5813999999999999;-3.6377999999999999;-3.6945000000000001;-3.7511999999999999;-3.8081;-3.8652000000000002;-3.9224999999999999]  InternalRulePriority=Speed  RndMeth=Simplest
  wheelbase_change vs wheel travel : Lookup_n-D  NumberOfTableDimensions=1  BreakpointsForDimension1=[-20;-19;-18;-17;-16;-15;-14;-13;-12;-11;-10;-9;-8;-7;-6;-5;-4;-3;-2;-1;0;1;2;3;4;5;6;7;8;9;10;11;12;13;14;15;16;17;18;19;20;21;22;23;24;25;26;27;28;29;30;31;32;33;34;35;36;37;38;39;40;41;42;43;44;45;46;47;48;49;50;51;52;53;54;55;56;57;58;59;60;61;62;63;64;65;66;67;68;69;70;71;72;73;74;75]  Table=[0.25;0.23999999999999999;0.22;0.20999999999999999;0.19;0.17999999999999999;0.16;0.14999999999999999;0.13;0.12;0.11;0.10000000000000001;0.080000000000000002;0.070000000000000007;0.059999999999999998;0.050000000000000003;0.040000000000000001;0.029999999999999999;0.02;0.01;0;-0.01;-0.02;-0.029999999999999999;-0.029999999999999999;-0.040000000000000001;-0.050000000000000003;-0.050000000000000003;-0.059999999999999998;-0.070000000000000007;-0.070000000000000007;-0.080000000000000002;-0.080000000000000002;-0.080000000000000002;-0.089999999999999997;-0.089999999999999997;-0.089999999999999997;-0.10000000000000001;-0.10000000000000001;-0.10000000000000001;-0.10000000000000001;-0.10000000000000001;-0.10000000000000001;-0.10000000000000001;-0.10000000000000001;-0.10000000000000001;-0.10000000000000001;-0.10000000000000001;-0.089999999999999997;-0.089999999999999997;-0.089999999999999997;-0.080000000000000002;-0.080000000000000002;-0.070000000000000007;-0.070000000000000007;-0.059999999999999998;-0.059999999999999998;-0.050000000000000003;-0.040000000000000001;-0.040000000000000001;-0.029999999999999999;-0.02;-0.01;0;0.01;0.02;0.029999999999999999;0.040000000000000001;0.050000000000000003;0.070000000000000007;0.080000000000000002;0.089999999999999997;0.11;0.12;0.13;0.14999999999999999;0.17000000000000001;0.17999999999999999;0.20000000000000001;0.22;0.23999999999999999;0.25;0.27000000000000002;0.28999999999999998;0.31;0.33000000000000002;0.34999999999999998;0.38;0.40000000000000002;0.41999999999999998;0.45000000000000001;0.46999999999999997;0.48999999999999999;0.52000000000000002;0.55000000000000004;0.56999999999999995]  InternalRulePriority=Speed  RndMeth=Simplest
  camber_FL : Outport
  h_ground_FL : Outport  Port=2
  delta_wb_FL : Outport  Port=3
  delta_z_tyre_FL : Outport  Port=4
  wires:
  Fz_FL/1 -> Front Left Tyre/4(Fz_FL)
  wheelbase_change vs wheel travel/1 -> Gain/1
  Delay One Step7/1 -> wheelbase_change vs wheel travel/1
  delta_Fz/1 -> Front Left Tyre/5(delta_Fz)
  Front Left Tyre/1(wheel_travel_FL) -> Delay One Step6/1, Delay One Step7/1, Delay One Step5/1, Delay One Step4/1
  Anti_dive vs wheel travel/1 -> Front Left Tyre/3(AD_FL)
  Front Left Tyre/2(h_ground_FL) -> h_ground_FL/1
  Delay One Step6/1 -> Anti_dive vs wheel travel/1
  IR vs wheel travel/1 -> Front Left Tyre/2(IR_FL)
  Delay One Step4/1 -> IR vs wheel travel/1
  Front Left Tyre/3(delta_z_tyre_FL) -> delta_z_tyre_FL/1
  Delay One Step5/1 -> camber vs wheel travel/1
  camber vs wheel travel/1 -> Add/2
  Constant/1 -> Add/1
  Add/1 -> camber_FL/1
  a/1 -> Front Left Tyre/6(a)
  car/1 -> Front Left Tyre/1(car)
  Gain/1 -> delta_wb_FL/1
